simulink model "ControlSystem"  (R2025b)
settings: Solver=VariableStepAuto  StartTime=0.0  StopTime=3  RelTol=1e-3
values from neighbouring files (symbols this model uses):
  Kc_val = double(sol.Kc(1))    [PID.m]
  Td_val = double(sol.Td(1))    [PID.m]
  Ti_val = double(sol.Ti(1))    [PID.m]
libraries: simulink x1
settings Model: Creator=mateo  LastModifiedBy=mateo

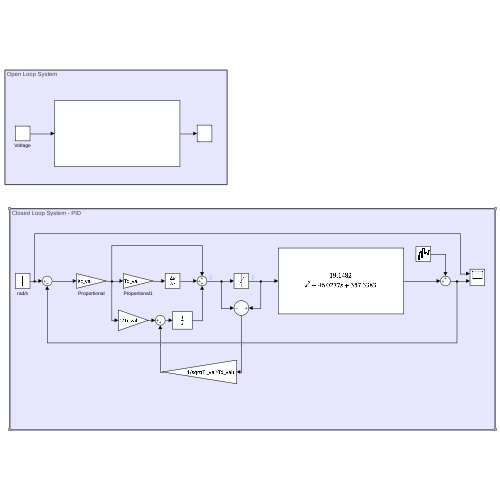
[thumbnail: Simulink's stored preview of the top-level diagram]
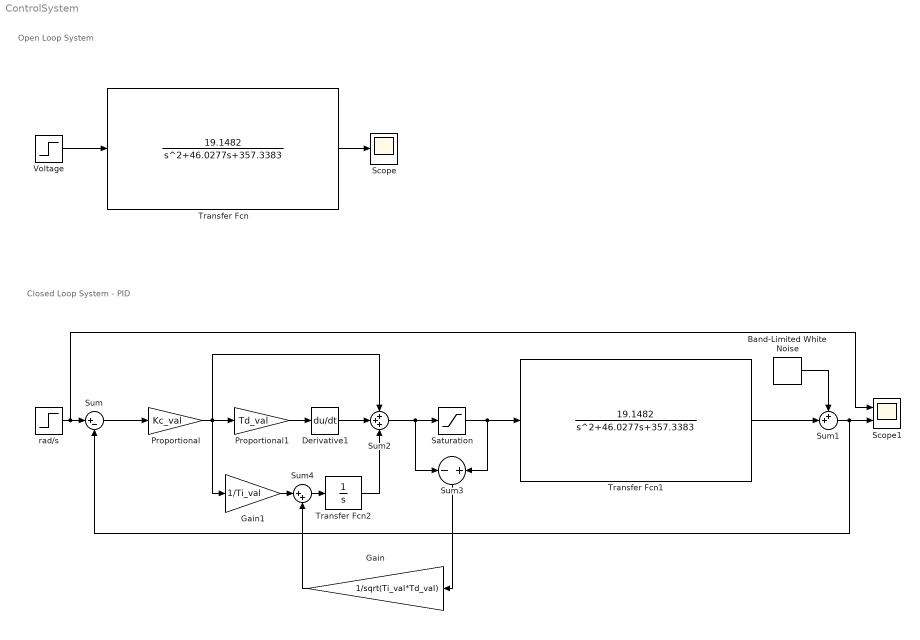
== system ControlSystem ==
  note: Open Loop System
  note: Closed Loop System - PID
  Band-Limited White Noise : simulink/Sources/Band-Limited White Noise  Cov=[1e-6]  Ts=0.1  seed=[23341]
  Derivative1 : Derivative
  Gain : Gain  Gain=1/sqrt(Ti_val*Td_val)
  Gain1 : Gain  Gain=1/Ti_val
  Proportional : Gain  Gain=Kc_val
  Proportional1 : Gain  Gain=Td_val
  Saturation : Saturate  UpperLimit=12  LowerLimit=0
  Scope : Scope
      settings: ActiveDisplayYMinimum=-0.0803784536949609  ActiveDisplayYMaximum=0.72340608325464817
  Scope1 : Scope  NumInputPorts=2
      settings: ActiveDisplayYMinimum=-0.0799534543561391  ActiveDisplayYMaximum=0.719581089205252
  Sum : Sum  Inputs=|+-
  Sum1 : Sum  Inputs=++|
  Sum2 : Sum  Inputs=+++
  Sum3 : Sum  Inputs=-+
  Sum4 : Sum  Inputs=|++
  Transfer Fcn : TransferFcn  Numerator=[19.1482]  Denominator=[1 46.0277 357.3383]
  Transfer Fcn1 : TransferFcn  Numerator=[19.1482]  Denominator=[1 46.0277 357.3383]
  Transfer Fcn2 : TransferFcn  Denominator=[1 0]
  Voltage : Step  Time=0.1  After=12  SampleTime=0
  rad/s : Step  Time=0.1  After=0.628319  SampleTime=0
  wires:
  Transfer Fcn/1 -> Scope/1
  Voltage/1 -> Transfer Fcn/1
  rad/s/1 -> Scope1/1, Sum/1
  Transfer Fcn1/1 -> Sum1/2
  Sum1/1 -> Sum/2, Scope1/2
  Sum/1 -> Proportional/1
  Proportional/1 -> Gain1/1, Proportional1/1, Sum2/1
  Sum2/1 -> Saturation/1, Sum3/1
  Saturation/1 -> Sum3/2, Transfer Fcn1/1
  Gain1/1 -> Sum4/1
  Sum4/1 -> Transfer Fcn2/1
  Gain/1 -> Sum4/2
  Sum3/1 -> Gain/1
  Derivative1/1 -> Sum2/2
  Proportional1/1 -> Derivative1/1
  Transfer Fcn2/1 -> Sum2/3
  Band-Limited White Noise/1 -> Sum1/1
